simulink model "AC_PCS_mo_2018a"  (R2018b)
settings: Solver=ode4  StartTime=0.0  StopTime=1.2  FixedStep=1e-6  RelTol=1e-3
undefined symbols (not defined in the file): Ion, Lithium
libraries: powerlib x29, powerlib_meascontrol x14, powerlib_extras x6, simulink x4, electricdrivelib x1, re_lib x1
settings Model: Creator=kc  LastModifiedBy=12657

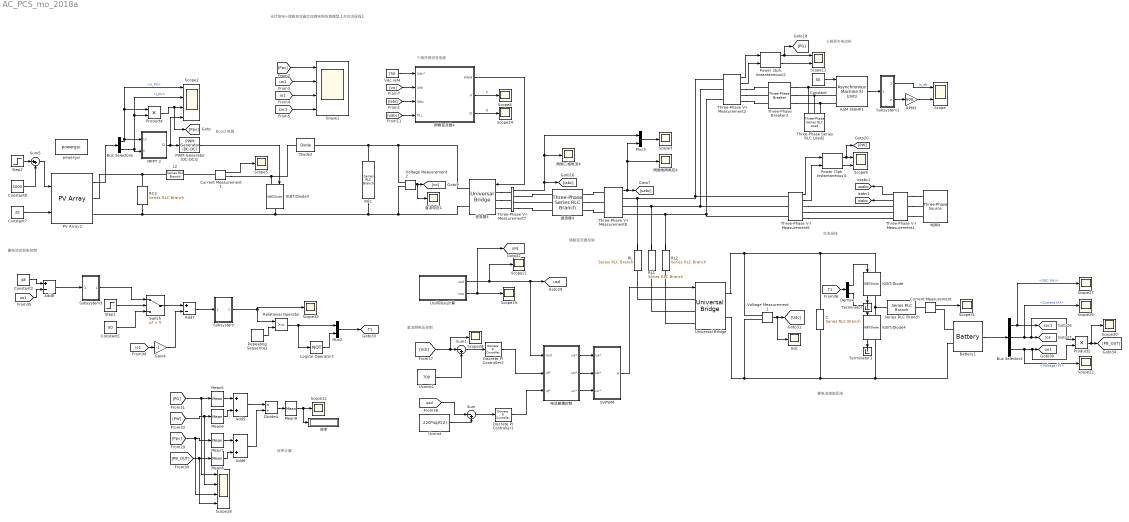
== system AC_PCS_mo_2018a ==
  note: 光伏发电+储能变流器交流微电网仿真模型【共交流母线】
  note: 蓄电池充放电控制
  note: 直流侧电压控制
  note: 三相并网逆变电路
  note: 蓄电池储能系统
  note: 效率计算
  note: 三相异步电动机
  note: 交流母线
  note: 储能变流器控制
  note: Boost 电路
  ASM 350HP1 : powerlib/Machines/Asynchronous Machine SI Units  RotorType=Squirrel-cage  PresetModel=No  MechanicalLoad=Torque Tm  ShowDetailedParameters=on  ReferenceFrame=Rotor  Units=SI  MeasurementBus=off  NominalParameters=[ 2250*746, 400, 50 ]  Stator=[ 0.029 0.226/377]  Rotor=[ 0.022 0.226/377]  Cage1=[ 0.022 0.226/377]  Cage2=[ 0.022 0.226/377]  Lm=13.04/377  Mechanical=[ 63.87 0 2]  PolePairs=2  InitialConditions=[0.00611928 0 556.114 556.114 556.114 -53.9807 -173.981 66.0193]  SimulateSaturation=off  Saturation=[14.03593122, 27.81365428, 53.79336849, 72.68890987, 97.98006896, 148.6815601, 215.7428561, 302.9841135, 428.7778367 ; 230, 322, 414, 460, 506, 552, 598, 644, 690]  LoadFlowParameters=1492000  TsPowergui=0  TsBlock=-1  IterativeModel=Forward Euler  IterativeDiscreteModel=Trapezoidal non iterative  Pmec=1.492e+006
      settings: SourceProductName=Simscape Electrical
  Add5 : Sum
  Add6 : Sum
  Add7 : Sum  Inputs=+-
  Add8 : Sum  Inputs=+-
  Battery1 : electricdrivelib/Extra Sources/Battery  BatType=Lithium-Ion  ShowTempParam=off  ThermalPreset=no  ShowAgeParam=off  NomV=48  NomQ=20  SOC=50  Batt_Tr=0.02  PresetModel=off  MaxQ=20  MinV=36  FullV=52  Dis_rate=8.6957  R=0.024  Normal_OP=18.087  expZone="[51.8585     0.982609]"  current=[6.5 13 32.5]  Units=Time  Tci=20  NomT=20  T2=-30  MaxQ2=4.8  FullV2=7.1  Normal_OP2=5.655  expZone2="[6.58           1]"  Rca=0.6  ti=2000  Dp=0  Neq0=0  Tsim=1e6  Ta1=25  Qeol=5.4*0.9  Reol=0.013333*1.2  Char_age=[2.3478, 3]  Dis_age=[2.3478, 10]  N1=1500  N2=10500  N3=1000  N4=1400  Ta2=45  N5=950
      settings: SourceProductName=Simscape Electrical
  Bus Selector2 : BusSelector  OutputSignals=SOC (%),Current (A),Voltage (V)
  Bus Selector6 : BusSelector  OutputSignals=V_PV,I_PV
  C : powerlib/Elements/Series RLC Branch  LConnTagsString=__new0  RConnTagsString=__new0  BranchType=C  Resistance=0.02  Inductance=4e-3  SetiL0=off  InitialCurrent=0  Capacitance=4e-3  Setx0=on  InitialVoltage=650  Measurements=None
      settings: SourceProductName=Simscape Electrical
  Constant : Constant  Value=50
  Constant1 : Constant  Value=50
  Constant2 : Constant  Value=48
  Constant7 : Constant  Value=25
  Constant8 : Constant  Value=1000
  Current Measurement : powerlib/Measurements/Current Measurement  PhasorSimulation=off  OutputType=Complex  PSBequivalent=0
      settings: SourceProductName=Simscape Electrical
  Current Measurement1 : powerlib/Measurements/Current Measurement  PhasorSimulation=off  OutputType=Complex  PSBequivalent=0
      settings: SourceProductName=Simscape Electrical
  Demux : Demux  Outputs=2
  Diode2 : powerlib/Power Electronics/Diode  Ron=0.001  Lon=0  Vf=0.8  IC=0  UseSnubber=off  Rs=500  Cs=250e-9  Measurements=off
      settings: SourceProductName=Simscape Electrical
  Discrete PI Controller1 : powerlib_extras/Discrete  Control Blocks/Discrete PI Controller  Kp=1.2  Ki=30  Par_Limits=[50000 -50000]  Init=0  Ts=1e-6
  Discrete PI Controller2 : powerlib_extras/Discrete  Control Blocks/Discrete PI Controller  Kp=1.2  Ki=90  Par_Limits=[50000 -50000]  Init=0  Ts=1e-6
  Divide4 : Product  Inputs=*/
  Gain4 : Gain  Gain=-1
  IGBT/Diode : powerlib/Power Electronics/IGBT//Diode  Ron=1e-3  Rs=1e5  Cs=inf  Measurements=on
      settings: SourceProductName=Simscape Electrical
  IGBT/Diode3 : powerlib/Power Electronics/IGBT//Diode  Ron=1e-3  Rs=1e5  Cs=inf  Measurements=off
      settings: SourceProductName=Simscape Electrical
  IGBT/Diode4 : powerlib/Power Electronics/IGBT//Diode  Ron=1e-3  Rs=1e5  Cs=inf  Measurements=on
      settings: SourceProductName=Simscape Electrical
  L2 : powerlib/Elements/Series RLC Branch  LConnTagsString=__new0  RConnTagsString=__new0  BranchType=L  Resistance=1  Inductance=6e-3  SetiL0=off  InitialCurrent=0  Capacitance=2e-4  Setx0=off  InitialVoltage=0  Measurements=None
      settings: SourceProductName=Simscape Electrical
  Logical Operator1 : Logic  Operator=NOT  AllPortsSameDT=off  OutDataTypeStr=boolean
  MPPT 2 : Subsystem  TreatAsAtomicUnit=on
  Mean5 : powerlib_meascontrol/Measurements/Mean  Freq=50  Vinit=0  Ts=1e-6
      settings: SourceProductName=Simscape Electrical
  Mean6 : powerlib_meascontrol/Measurements/Mean  Freq=50  Vinit=0  Ts=1e-6
      settings: SourceProductName=Simscape Electrical
  Mean7 : powerlib_meascontrol/Measurements/Mean  Freq=50  Vinit=10  Ts=1e-6
      settings: SourceProductName=Simscape Electrical
  Mean8 : powerlib_meascontrol/Measurements/Mean  Freq=50  Vinit=10  Ts=1e-6
      settings: SourceProductName=Simscape Electrical
  Mean9 : powerlib_meascontrol/Measurements/Mean  Freq=50  Vinit=10  Ts=1e-6
      settings: SourceProductName=Simscape Electrical
  Mux2 : Mux  Inputs=2
  Mux3 : Mux  Inputs=2
  PV Array2 : re_lib/Solar/PV Array  Npar=5  Nser=10  PlotType=array @ 25 deg.C & specified irradiances  S_vec="[ 1000  500  100 ]"  Temp_C_vec="[ 45 25  ]"  ModuleName=A10Green Technology A10J-M60-230  PlotWhenSelected=off  Pm=230.1288  Ncell=60  Voc=36.42  Isc=8.1  Vm=30.36  Im=7.58  beta_Voc_pc=-0.35901  alpha_Isc_pc=0.097  beta_Voc=-0.13075  alpha_Isc=0.007857  IL=8.1068  I0=2.792e-10  nI=0.98145  Rsh=234.4496  Rs=0.19818  BAL=off  Tc=1e-6  Tfilter=5e-5
      settings: SourceProductName=Simscape Electrical
  PWM Generator (DC-DC)2 : powerlib_meascontrol/Pulse & Signal Generators/PWM Generator (DC-DC)  Fsw=20000  Ts=0
      settings: SourceProductName=Simscape Electrical
  "Power (3ph, Instantaneous)1" : powerlib_meascontrol/Measurements/Power (3ph, Instantaneous)
      settings: SourceProductName=Simscape Electrical
  "Power (3ph, Instantaneous)2" : powerlib_meascontrol/Measurements/Power (3ph, Instantaneous)
      settings: SourceProductName=Simscape Electrical
  Product2 : Product
  Product4 : Product
  RC1 : powerlib/Elements/Series RLC Branch  LConnTagsString=__new0  RConnTagsString=__new0  BranchType=C  Resistance=0.001  Inductance=1e-3  SetiL0=off  InitialCurrent=0  Capacitance=3e-2  Setx0=on  InitialVoltage=750  Measurements=None
      settings: SourceProductName=Simscape Electrical
  RC3 : powerlib/Elements/Series RLC Branch  LConnTagsString=__new0  RConnTagsString=__new0  BranchType=C  Resistance=0.1  Inductance=1e-3  SetiL0=off  InitialCurrent=0  Capacitance=1e-3  Setx0=on  InitialVoltage=300  Measurements=None
      settings: SourceProductName=Simscape Electrical
  RL : powerlib/Elements/Series RLC Branch  LConnTagsString=__new0  RConnTagsString=__new0  BranchType=RL  Resistance=0.02  Inductance=2e-3  SetiL0=off  InitialCurrent=0  Capacitance=1e-6  Setx0=off  InitialVoltage=0  Measurements=None
      settings: SourceProductName=Simscape Electrical
  RL1 : powerlib/Elements/Series RLC Branch  LConnTagsString=__new0  RConnTagsString=__new0  BranchType=RL  Resistance=0.02  Inductance=2e-3  SetiL0=off  InitialCurrent=0  Capacitance=1e-6  Setx0=off  InitialVoltage=0  Measurements=None
      settings: SourceProductName=Simscape Electrical
  RL2 : powerlib/Elements/Series RLC Branch  LConnTagsString=__new0  RConnTagsString=__new0  BranchType=RL  Resistance=0.02  Inductance=2e-3  SetiL0=off  InitialCurrent=0  Capacitance=1e-6  Setx0=off  InitialVoltage=0  Measurements=None
      settings: SourceProductName=Simscape Electrical
  RPM3 : Gain  Gain=500  SaturateOnIntegerOverflow=on  OutDataTypeStr=Inherit: Same as input  ParamDataTypeStr=Inherit: Same as input
  Relational Operator : RelationalOperator  OutDataTypeStr=boolean  RndMeth=Simplest
  Repeating Sequence1 : simulink/Sources/Repeating Sequence  rep_seq_t=[0 0.025e-3 0.05e-3]  rep_seq_y=[0 1 0]
  SVPWM : Subsystem
  Scope : Scope  NumInputPorts=2
  Scope1 : Scope  NumInputPorts=4
  Scope11 : Scope  NumInputPorts=2
  Scope{3,5,8,12,19,21..22,24,27..32} (14 alike) : Scope
  Scope18 : Scope  NumInputPorts=4
  Scope2 : Scope  NumInputPorts=4
  Scope9 : Scope  NumInputPorts=2
  Series RLC Branch : powerlib/Elements/Series RLC Branch  LConnTagsString=__new0  RConnTagsString=__new0  BranchType=L  Resistance=1  Inductance=1e-3  SetiL0=off  InitialCurrent=0  Capacitance=1e-6  Setx0=off  InitialVoltage=0  Measurements=None
      settings: SourceProductName=Simscape Electrical
  Step1 : Step  Time=0  SampleTime=0
  Step2 : Step  Time=2  After=200  SampleTime=0
  Subsystem : Subsystem
      mask Display: disp('PI')
  Subsystem1 : Subsystem
  Subsystem3 : Subsystem
      mask Display: disp('PI')
  Sum : Sum  Inputs=|-+
  Sum1 : Sum  Inputs=|-+
  Sum5 : Sum  Inputs=|++
  Switch : Switch  Criteria=u2 > Threshold
  Terminator : Terminator
  Terminator1 : Terminator
  Three-Phase Series RLC Load2 : powerlib/Elements/Three-Phase Series RLC Load  LConnTagsString=A|B|C  Configuration=Y (grounded)  NominalVoltage=380  Vabc=[1e3 1e3 1e3]  Vabcp=[1e3 1e3 1e3]  NominalFrequency=50  UnbalancedPower=off  ActivePower=5e2  InductivePower=0  CapacitivePower=0  Pabc=[10e3 9e3 11e3]  QLabc=[100 90 110]  QCabc=[100 90 110]  Pabcp=[10e3 9e3 11e3]  QLabcp=[100 90 110]  QCabcp=[100 90 110]  Measurements=None  LoadType=constant Z
      settings: SourceProductName=Simscape Electrical
  Three-Phase V-I Measurement1 : powerlib/Measurements/Three-Phase V-I Measurement  VoltageMeasurement=phase-to-ground  SetLabelV=off  LabelV=Vabc  Vpu=off  VpuLL=off  CurrentMeasurement=yes  SetLabelI=off  LabelI=Iabc  Ipu=off  Pbase=100e6  Vbase=500e3  OutputType=Complex  PhasorSimulation=off  PSBequivalent=0
      settings: SourceProductName=Simscape Electrical
  Three-Phase V-I Measurement2 : powerlib/Measurements/Three-Phase V-I Measurement  VoltageMeasurement=phase-to-ground  SetLabelV=off  LabelV=uabc  Vpu=off  VpuLL=off  CurrentMeasurement=yes  SetLabelI=off  LabelI=iabc1  Ipu=off  Pbase=100e6  Vbase=500e3  OutputType=Complex  PhasorSimulation=off  PSBequivalent=0
      settings: SourceProductName=Simscape Electrical
  Three-Phase V-I Measurement5 : powerlib/Measurements/Three-Phase V-I Measurement  VoltageMeasurement=phase-to-ground  SetLabelV=off  LabelV=Vabc  Vpu=off  VpuLL=off  CurrentMeasurement=yes  SetLabelI=off  LabelI=Iabc  Ipu=off  Pbase=100e6  Vbase=500e3  OutputType=Complex  PhasorSimulation=off  PSBequivalent=0
      settings: SourceProductName=Simscape Electrical
  Three-Phase V-I Measurement7 : powerlib/Measurements/Three-Phase V-I Measurement  VoltageMeasurement=no  SetLabelV=off  LabelV=Vabc  Vpu=off  VpuLL=off  CurrentMeasurement=yes  SetLabelI=off  LabelI=iabc  Ipu=off  Pbase=100e6  Vbase=500e3  OutputType=Complex  PhasorSimulation=off  PSBequivalent=0
      settings: SourceProductName=Simscape Electrical
  Three-Phase V-I Measurement8 : powerlib/Measurements/Three-Phase V-I Measurement  VoltageMeasurement=phase-to-ground  SetLabelV=off  LabelV=uabc  Vpu=off  VpuLL=off  CurrentMeasurement=no  SetLabelI=on  LabelI=iabc1  Ipu=off  Pbase=100e6  Vbase=500e3  OutputType=Complex  PhasorSimulation=off  PSBequivalent=0
      settings: SourceProductName=Simscape Electrical
  Three-Phase Breaker2 : powerlib/Elements/Three-Phase Breaker  InitialState=open  SwitchA=on  SwitchB=on  SwitchC=on  SwitchTimes=[0]  External=off  BreakerResistance=0.01  SnubberResistance=1e6  SnubberCapacitance=inf  Measurements=None
      settings: SourceProductName=Simscape Electrical
  Uconst : Constant  Value=220*sqrt(2)
  Uconst1 : Constant  Value=700
  Udc : Scope
  Universal Bridge : powerlib/Power Electronics/Universal Bridge  Arms=3  SnubberResistance=1e5  SnubberCapacitance=inf  Device=IGBT / Diodes  Ron=1e-3  Lon=0  ForwardVoltages="[  0  0  ]"  ForwardVoltage=0  GTOparameters=[ 10e-6 , 20e-6 ]  IGBTparameters=[ 1e-6 , 2e-6 ]  Measurements=None  Measurements_2=None  converterType=Rectifier
      settings: SourceProductName=Simscape Electrical
  Usd和Usq计算 : Subsystem
  Vdc,ref4 : Constant  Value=750
  Voltage Measurement1 : powerlib/Measurements/Voltage Measurement  PhasorSimulation=off  OutputType=Complex  PSBequivalent=0
      settings: SourceProductName=Simscape Electrical
  Voltage Measurement2 : powerlib/Measurements/Voltage Measurement  PhasorSimulation=off  OutputType=Complex  PSBequivalent=0
      settings: SourceProductName=Simscape Electrical
  powergui : powerlib/powergui  Priority=1  SimulationMode=Discrete  SampleTime=1e-6  frequency=60  Iterations=50  frequencyindice=0  Pbase=100e6  ErrMax=1e-4  UnitsV=kV  UnitsW=MW  buscounter=0  FunctionMessages=off  echomessages=off  EnableUseOfTLC=off  CurrentSourceSwitches=off  DisableSnubberDevices=off  DisableRonSwitches=off  DisableVfSwitches=off  DisplayEquations=off  SolverType=Tustin/Backward Euler (TBE)  Interpol=off  ExternalGateDelay=off  methode=off  Ts=100  x0status=blocks  SPID=on  SwTol=0  HookPort=off  RestoreLinks=warning  ResistiveCurrentMeasurement=off  Frange=[0:2:500]  Ylog=off  Xlog=on  ShowGrid=off  save=off  variable=ZData  structure=0  ZoomFFT=off  StartTime=0.0  cycles=1  DisplayStyle=1  fundamental=60  FreqAxis=off  MaxFrequency=1000  frequencyindicesteady=1  RmsSteady=1  display=off
  效率 : Display
  滤波器4 : powerlib/Elements/Three-Phase Series RLC Branch  LConnTagsString=A|B|C  RConnTagsString=A|B|C  BranchType=RL  Resistance=3/8  Inductance=8e-3  Capacitance=1e-6  Measurements=None
      settings: SourceProductName=Simscape Electrical
  电流解耦控制 : Subsystem
  电网4 : powerlib/Electrical Sources/Three-Phase Source  InternalConnection=Yg  VoltagePhases=off  Voltage=380  PhaseAngle=0  Voltage_phases=[25e3 25e3 25e3]/sqrt(3)  PhaseAngles_phases=[0 -120 +120]  Frequency=50  NonIdealSource=off  SpecifyImpedance=off  Resistance=0.01  Inductance=0  ShortCircuitLevel=100e6  BaseVoltage=25e3  XRratio=7  BusType=swing  Pref=0  Qref=0  Prefabc=[10e3, 10e3, 10e3]  Qrefabc=[0, 0, 0]  Qmin=-inf  Qmax=inf
      settings: SourceProductName=Simscape Electrical
  直流电压1 : Scope
  网侧三相电流4 : Scope
  网侧变流器4 : Subsystem
  网侧电网电压4 : Scope
  逆变器4 : powerlib/Power Electronics/Universal Bridge  Arms=3  SnubberResistance=1e5  SnubberCapacitance=inf  Device=IGBT / Diodes  Ron=1e-3  Lon=0  ForwardVoltages="[  0  0  ]"  ForwardVoltage=0  GTOparameters=[ 10e-6 , 20e-6 ]  IGBTparameters=[ 5e-6 , 5e-6 ]  Measurements=None  Measurements_2=None  converterType=Rectifier
      settings: SourceProductName=Simscape Electrical
  tag scope: T1=global, io1=global, isabc=global, soc1=global, uo1=global, usabc=global, usd=global, usq=global
  wires:
  Three-Phase V-I Measurement8/1 -> Mux3/2, 网侧电网电压4/1, [uabc]
  Mux3/1 -> Scope3/1
  [uabc] -> 网侧变流器4/4(PLL)
  网侧变流器4/2(P) -> Scope8/1  "P"
  网侧变流器4/3(Q) -> Scope24/1  "Q"
  [iabc] -> 网侧变流器4/3(Iabc)
  网侧变流器4/1(PWM) -> 逆变器4/1
  [vo] -> 网侧变流器4/2(Udc)
  Vdc,ref4/1 -> 网侧变流器4/1(Udc*)
  Three-Phase V-I Measurement7/1 -> Mux3/1, 网侧三相电流4/1, [iabc]
  Constant/1 -> ASM 350HP1/1
  Three-Phase V-I Measurement1/1 -> [usabc]
  Three-Phase V-I Measurement1/2 -> [isabc]
  ASM 350HP1/1 -> Subsystem1/1(In1)
  Subsystem1/1(is_ab) -> Scope/1  "is_ab"
  RPM3/1 -> Scope/2
  Subsystem1/2(w) -> RPM3/1
  "Power (3ph, Instantaneous)1"/1 -> [PW], Scope9/1
  "Power (3ph, Instantaneous)1"/2 -> Scope9/2
  Three-Phase V-I Measurement2/1 -> "Power (3ph, Instantaneous)2"/1
  Three-Phase V-I Measurement2/2 -> "Power (3ph, Instantaneous)2"/2
  "Power (3ph, Instantaneous)2"/1 -> [PG], Scope11/1
  "Power (3ph, Instantaneous)2"/2 -> Scope11/2
  Three-Phase V-I Measurement5/1 -> "Power (3ph, Instantaneous)1"/1
  Three-Phase V-I Measurement5/2 -> "Power (3ph, Instantaneous)1"/2
  Add5/1 -> Divide4/1
  Divide4/1 -> Mean9/1
  Add6/1 -> Divide4/2
  Mean5/1 -> Add5/1
  [PG] -> Scope18/1, Mean5/1
  [PW] -> Scope18/2, Mean6/1
  Mean6/1 -> Add5/2
  Mean7/1 -> Add6/1
  [Ppv] -> Scope18/3, Mean7/1
  [PB_OUT] -> Scope18/4, Mean8/1
  Mean8/1 -> Add6/2
  Mean9/1 -> 效率/1, Scope12/1
  [Udc] -> Scope28/1, Sum1/1
  Sum1/1 -> Discrete PI Controller2/1
  Uconst1/1 -> Sum1/2
  Discrete PI Controller2/1 -> 电流解耦控制/2(id*)
  Constant2/1 -> Add8/1
  [io1] -> Gain4/1
  Constant1/1 -> Switch/3
  Gain4/1 -> Add7/2
  Logical Operator1/1 -> Mux2/2
  Switch/1 -> Add7/1
  Mux2/1 -> [T1]
  Subsystem/1(Out1) -> Scope32/1, Relational Operator/1
  Add8/1 -> Subsystem3/1(In1)
  Add7/1 -> Subsystem/1(In1)
  Subsystem3/1(Out1) -> Switch/1
  Repeating Sequence1/1 -> Relational Operator/2
  [uo1] -> Add8/2
  Step1/1 -> Switch/2
  Relational Operator/1 -> Mux2/1, Logical Operator1/1
  Product2/1 -> Scope30/1, [PB_OUT]
  电流解耦控制/2(ub*) -> SVPWM/2(ub*)
  [usd] -> Sum/1
  [T1] -> Demux/1
  Voltage Measurement1/1 -> [Udc], Udc/1
  Demux/2 -> IGBT/Diode4/1
  Demux/1 -> IGBT/Diode/1
  IGBT/Diode4/1 -> Terminator1/1
  Battery1/1 -> Bus Selector2/1
  Bus Selector2/1 -> Scope27/1, [soc1]  "<SOC (%)>"
  Bus Selector2/3 -> Scope22/1, Product2/2, [uo1]  "<Voltage (V)>"
  IGBT/Diode/1 -> Terminator/1
  Discrete PI Controller1/1 -> 电流解耦控制/3(iq*)
  Usd和Usq计算/2(usq) -> [usq], Scope19/1
  Bus Selector2/2 -> Scope29/1, Product2/1, [io1]  "<Current (A)>"
  Uconst/1 -> Sum/2
  电流解耦控制/1(ua*) -> SVPWM/1(ua*)
  Current Measurement/1 -> Scope31/1
  Usd和Usq计算/1(usd) -> [usd], 电流解耦控制/1(Usd), Scope21/1
  电流解耦控制/3(uc*) -> SVPWM/3(uc*)
  SVPWM/1(g) -> Universal Bridge/1
  Sum/1 -> Discrete PI Controller1/1
  [Ppv] -> Scope1/1
  [uo1] -> Scope1/2
  [io1] -> Scope1/3
  [soc1] -> Scope1/4
  Bus Selector6/1 -> Product4/1, Scope2/1, MPPT 2/1("Ui ")  "<V_PV>"
  PWM Generator (DC-DC)2/1 -> IGBT/Diode3/1
  Constant8/1 -> Sum5/2
  PV Array2/1 -> Bus Selector6/1
  Sum5/1 -> PV Array2/1
  Bus Selector6/2 -> Product4/2, Scope2/2, MPPT 2/2("Ii ")  "<I_PV>"
  Step2/1 -> Sum5/1
  Product4/1 -> [Ppv], Scope2/3
  Constant7/1 -> PV Array2/2
  MPPT 2/1(D) -> Scope2/4, PWM Generator (DC-DC)2/1
  Current Measurement1/1 -> Scope5/1
  Voltage Measurement2/1 -> [vo], 直流电压1/1
  connections:
  逆变器4/LConn2 -- Three-Phase V-I Measurement7/LConn2
  逆变器4/LConn3 -- Three-Phase V-I Measurement7/LConn3
  滤波器4/RConn2 -- Three-Phase V-I Measurement8/LConn2
  滤波器4/RConn1 -- Three-Phase V-I Measurement8/LConn1
  Three-Phase V-I Measurement7/RConn1 -- 滤波器4/LConn1
  滤波器4/RConn3 -- Three-Phase V-I Measurement8/LConn3
  逆变器4/LConn1 -- Three-Phase V-I Measurement7/LConn1
  滤波器4/LConn2 -- Three-Phase V-I Measurement7/RConn2
  Three-Phase V-I Measurement7/RConn3 -- 滤波器4/LConn3
  Three-Phase Series RLC Load2/LConn1 -- Three-Phase Breaker2/RConn1 -- ASM 350HP1/LConn1
  Three-Phase Series RLC Load2/LConn2 -- Three-Phase Breaker2/RConn2 -- ASM 350HP1/LConn2
  Three-Phase Series RLC Load2/LConn3 -- ASM 350HP1/LConn3 -- Three-Phase Breaker2/RConn3
  Three-Phase V-I Measurement1/LConn1 -- 电网4/RConn1
  Three-Phase V-I Measurement1/LConn2 -- 电网4/RConn2
  Three-Phase V-I Measurement1/LConn3 -- 电网4/RConn3
  Three-Phase V-I Measurement2/RConn1 -- Three-Phase Breaker2/LConn1
  Three-Phase V-I Measurement2/RConn2 -- Three-Phase Breaker2/LConn2
  Three-Phase V-I Measurement2/RConn3 -- Three-Phase Breaker2/LConn3
  Three-Phase V-I Measurement5/RConn1 -- Three-Phase V-I Measurement1/RConn1
  Three-Phase V-I Measurement5/RConn2 -- Three-Phase V-I Measurement1/RConn2
  Three-Phase V-I Measurement5/RConn3 -- Three-Phase V-I Measurement1/RConn3
  C/RConn1 -- IGBT/Diode4/RConn1 -- Battery1/LConn2 -- Universal Bridge/RConn2 -- Voltage Measurement1/LConn2
  Universal Bridge/RConn1 -- Voltage Measurement1/LConn1 -- C/LConn1 -- IGBT/Diode/LConn1
  IGBT/Diode/RConn1 -- Series RLC Branch/LConn1 -- IGBT/Diode4/LConn1
  Current Measurement/LConn1 -- Series RLC Branch/RConn1
  Battery1/LConn1 -- Current Measurement/RConn1
  Universal Bridge/LConn3 -- RL2/RConn1
  Universal Bridge/LConn2 -- RL1/RConn1
  Universal Bridge/LConn1 -- RL/RConn1
  Three-Phase V-I Measurement8/RConn1 -- Three-Phase V-I Measurement5/LConn1 -- Three-Phase V-I Measurement2/LConn1 -- RL/LConn1
  Three-Phase V-I Measurement8/RConn2 -- Three-Phase V-I Measurement2/LConn2 -- Three-Phase V-I Measurement5/LConn2 -- RL1/LConn1
  RL2/LConn1 -- Three-Phase V-I Measurement2/LConn3 -- Three-Phase V-I Measurement5/LConn3 -- Three-Phase V-I Measurement8/RConn3
  L2/LConn1 -- PV Array2/RConn1 -- RC3/LConn1
  PV Array2/RConn2 -- RC1/RConn1 -- Voltage Measurement2/LConn2 -- 逆变器4/RConn2 -- IGBT/Diode3/RConn1 -- RC3/RConn1
  Current Measurement1/RConn1 -- IGBT/Diode3/LConn1 -- Diode2/LConn1
  RC1/LConn1 -- Diode2/RConn1 -- 逆变器4/RConn1 -- Voltage Measurement2/LConn1
  Current Measurement1/LConn1 -- L2/RConn1

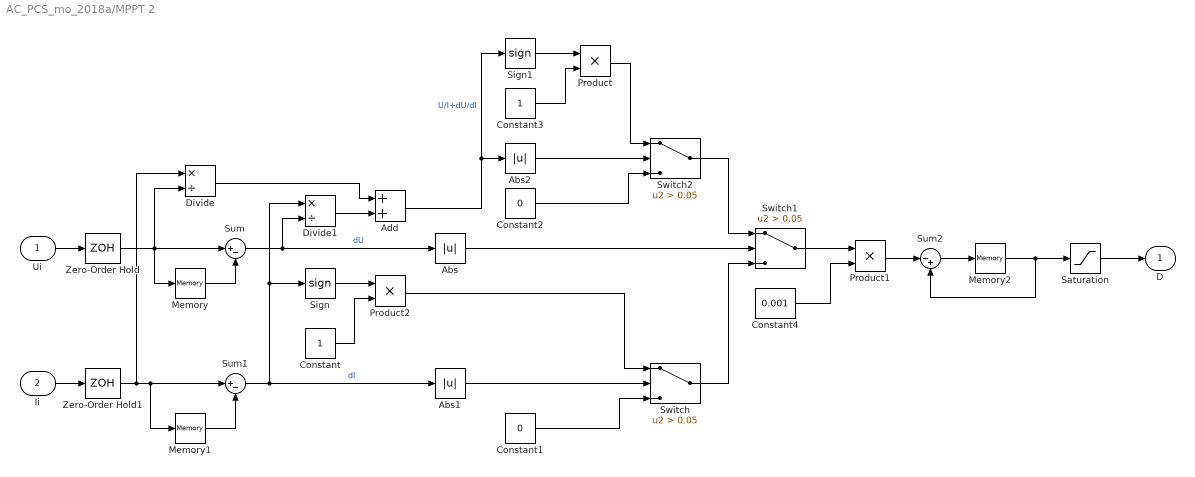
== system AC_PCS_mo_2018a/MPPT 2 ==
  "Ui " : Inport
  "Ii " : Inport  Port=2
  Abs : Abs
  Abs1 : Abs
  Abs2 : Abs
  Add : Sum
  Constant : Constant
  Constant1 : Constant  Value=0
  Constant2 : Constant  Value=0
  Constant3 : Constant
  Constant4 : Constant  Value=0.001
  Divide : Product  Inputs=*/
  Divide1 : Product  Inputs=*/
  Memory : Memory  InheritSampleTime=on
  Memory1 : Memory  InheritSampleTime=on
  Memory2 : Memory  InitialCondition=0.6  InheritSampleTime=on
  Product : Product
  Product1 : Product
  Product2 : Product
  Saturation : Saturate  UpperLimit=1  LowerLimit=0
  Sign : Signum
  Sign1 : Signum
  Sum : Sum  Inputs=|+-
  Sum1 : Sum  Inputs=|+-
  Sum2 : Sum  Inputs=|-+
  Switch : Switch  Criteria=u2 > Threshold  Threshold=0.05
  Switch1 : Switch  Criteria=u2 > Threshold  Threshold=0.05
  Switch2 : Switch  Criteria=u2 > Threshold  Threshold=0.05
  Zero-Order Hold : ZeroOrderHold  SampleTime=0.01
  Zero-Order Hold1 : ZeroOrderHold  SampleTime=0.01
  D : Outport  VectorParamsAs1DForOutWhenUnconnected=on
  wires:
  "Ui "/1 -> Zero-Order Hold/1
  "Ii "/1 -> Zero-Order Hold1/1
  Zero-Order Hold/1 -> Sum/1, Divide/2, Memory/1
  Memory/1 -> Sum/2
  Memory1/1 -> Sum1/2
  Zero-Order Hold1/1 -> Sum1/1, Memory1/1, Divide/1
  Sum/1 -> Divide1/2, Abs/1  "dU"
  Sum1/1 -> Abs1/1, Sign/1, Divide1/1  "dI"
  Divide/1 -> Add/1
  Divide1/1 -> Add/2
  Sign/1 -> Product2/1
  Constant/1 -> Product2/2
  Abs1/1 -> Switch/2
  Constant1/1 -> Switch/3
  Product2/1 -> Switch/1
  Abs/1 -> Switch1/2
  Add/1 -> Abs2/1, Sign1/1  "U/I+dU/dI"
  Abs2/1 -> Switch2/2
  Constant2/1 -> Switch2/3
  Sign1/1 -> Product/1
  Constant3/1 -> Product/2
  Product/1 -> Switch2/1
  Switch2/1 -> Switch1/1
  Switch1/1 -> Product1/1
  Constant4/1 -> Product1/2
  Product1/1 -> Sum2/1
  Sum2/1 -> Memory2/1
  Memory2/1 -> Saturation/1, Sum2/2
  Saturation/1 -> D/1
  Switch/1 -> Switch1/3

== system AC_PCS_mo_2018a/SVPWM ==
  ua* : Inport
  ub* : Inport  Port=2
  uc* : Inport  Port=3
  Demux : Demux  Outputs=3
  Mux2 : Mux  Inputs=3
  Terminator : Terminator
  abc to Alpha-Beta-Zero : powerlib_meascontrol/Transformations/abc to Alpha-Beta-Zero
      settings: SourceProductName=Simscape Electrical
  svpwm1 : Subsystem
  g : Outport
  wires:
  ua*/1 -> Mux2/1
  Mux2/1 -> abc to Alpha-Beta-Zero/1
  ub*/1 -> Mux2/2
  uc*/1 -> Mux2/3
  abc to Alpha-Beta-Zero/1 -> Demux/1
  Demux/1 -> svpwm1/1(Ualfa)
  Demux/2 -> svpwm1/2(Ubeta)
  svpwm1/1(sb) -> g/1
  Demux/3 -> Terminator/1

== system AC_PCS_mo_2018a/Subsystem ==
  In1 : Inport
  Add1 : Sum
  Gain : Gain  Gain=20
  Gain1 : Gain  Gain=8
  Integrator : Integrator
  Out1 : Outport
  wires:
  In1/1 -> Gain1/1, Gain/1
  Gain1/1 -> Integrator/1
  Integrator/1 -> Add1/2
  Add1/1 -> Out1/1
  Gain/1 -> Add1/1

== system AC_PCS_mo_2018a/Subsystem1 ==
  In1 : Inport
  Bus Selector1 : BusSelector  OutputSignals=Stator measurements.Stator current is_a (A),Stator measurements.Stator current is_b (A),Stator measurements.Stator current is_c (A),Mechanical.Rotor speed (wm)
  Mux : Mux  Inputs=3
  rad/s to : Gain  Gain=60/2/pi  SaturateOnIntegerOverflow=on  OutDataTypeStr=Inherit: Same as input  ParamDataTypeStr=Inherit: Same as input
  is_ab : Outport  VectorParamsAs1DForOutWhenUnconnected=on
  w : Outport  Port=2  VectorParamsAs1DForOutWhenUnconnected=on
  wires:
  rad/s to/1 -> w/1  "Speed (rpm)"
  In1/1 -> Bus Selector1/1
  Bus Selector1/4 -> rad/s to/1  "<Rotor speed (wm)>"
  Bus Selector1/1 -> Mux/1  "<Stator current is_a (A)>"
  Bus Selector1/2 -> Mux/2  "<Stator current is_b (A)>"
  Bus Selector1/3 -> Mux/3  "<Stator current is_c (A)>"
  Mux/1 -> is_ab/1

== system AC_PCS_mo_2018a/Subsystem3 ==
  In1 : Inport
  Add5 : Sum
  Gain1 : Gain  Gain=10
  Gain5 : Gain  Gain=200
  Integrator2 : Integrator
  Out1 : Outport
  wires:
  Add5/1 -> Out1/1
  Gain1/1 -> Add5/1
  In1/1 -> Gain1/1, Gain5/1
  Gain5/1 -> Integrator2/1
  Integrator2/1 -> Add5/2

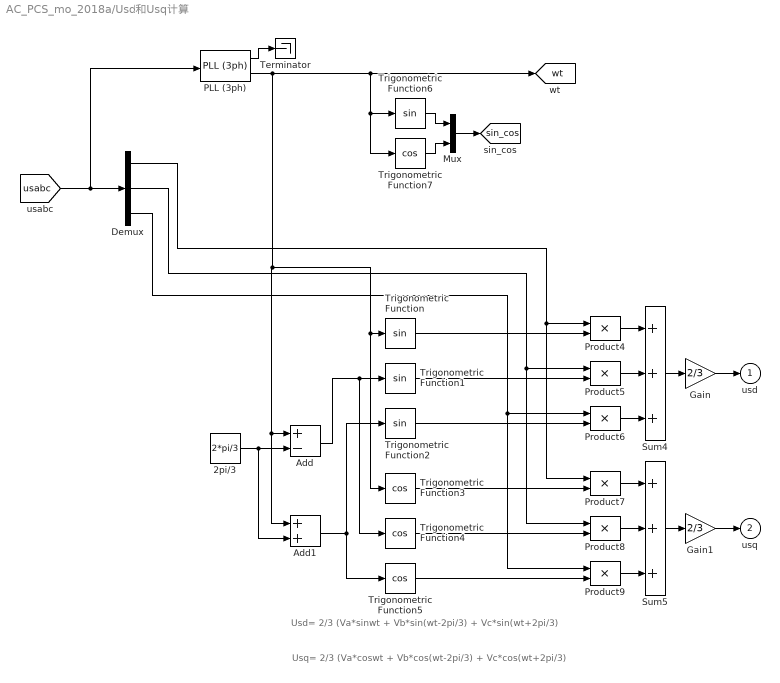
== system AC_PCS_mo_2018a/Usd和Usq计算 ==
  note: Usq= 2/3 (Va*coswt + Vb*cos(wt-2pi/3) + Vc*cos(wt+2pi/3)
  note: Usd= 2/3 (Va*sinwt + Vb*sin(wt-2pi/3) + Vc*sin(wt+2pi/3)
  2pi/3 : Constant  Value=2*pi/3
  Add : Sum  Inputs=+-
  Add1 : Sum
  Demux : Demux  Outputs=3
  Gain : Gain  Gain=2/3
  Gain1 : Gain  Gain=2/3
  Mux : Mux  Inputs=2
  PLL (3ph) : powerlib_meascontrol/PLL/PLL (3ph)  Fmin=45  Par_Init=[0, 50]  ParK=[180, 3200, 1]  TcD=1e-4  MaxRateChangeFreq=12  FilterCutOffFreq=25  Ts=1e-6  AGC=on
      settings: SourceProductName=Simscape Electrical
  Product{4..9} (6 alike) : Product  SaturateOnIntegerOverflow=on  InputSameDT=on  OutDataTypeStr=Inherit: Same as first input
  Sum4 : Sum  Inputs=+++  SaturateOnIntegerOverflow=on  InputSameDT=on  OutDataTypeStr=Inherit: Same as first input
  Sum5 : Sum  Inputs=+++  SaturateOnIntegerOverflow=on  InputSameDT=on  OutDataTypeStr=Inherit: Same as first input
  Terminator : Terminator
  Trigonometric Function{,1..2,6} (4 alike) : Trigonometry
  Trigonometric Function{3..5,7} (4 alike) : Trigonometry  Operator=cos
  usd : Outport  InitialOutput=0
  usq : Outport  Port=2  InitialOutput=0
  tag scope: sin_cos=global, wt=global
  wires:
  Mux/1 -> [sin_cos]
  PLL (3ph)/2 -> Add1/1, Add/1, Trigonometric Function/1, Trigonometric Function3/1, Trigonometric Function7/1, Trigonometric Function6/1, [wt]
  Trigonometric Function5/1 -> Product9/2
  Trigonometric Function4/1 -> Product8/2
  Trigonometric Function3/1 -> Product7/2
  Demux/3 -> Product6/1, Product9/1
  Trigonometric Function2/1 -> Product6/2
  Add1/1 -> Trigonometric Function2/1, Trigonometric Function5/1
  Demux/2 -> Product5/1, Product8/1
  Trigonometric Function1/1 -> Product5/2
  Add/1 -> Trigonometric Function1/1, Trigonometric Function4/1
  Trigonometric Function/1 -> Product4/2
  2pi/3/1 -> Add/2, Add1/2
  Sum5/1 -> Gain1/1
  Product8/1 -> Sum5/2
  Product9/1 -> Sum5/3
  Product7/1 -> Sum5/1
  Sum4/1 -> Gain/1
  Product4/1 -> Sum4/1
  Product6/1 -> Sum4/3
  Product5/1 -> Sum4/2
  Demux/1 -> Product4/1, Product7/1
  [usabc] -> PLL (3ph)/1, Demux/1
  PLL (3ph)/1 -> Terminator/1
  Trigonometric Function6/1 -> Mux/1
  Trigonometric Function7/1 -> Mux/2
  Gain/1 -> usd/1
  Gain1/1 -> usq/1

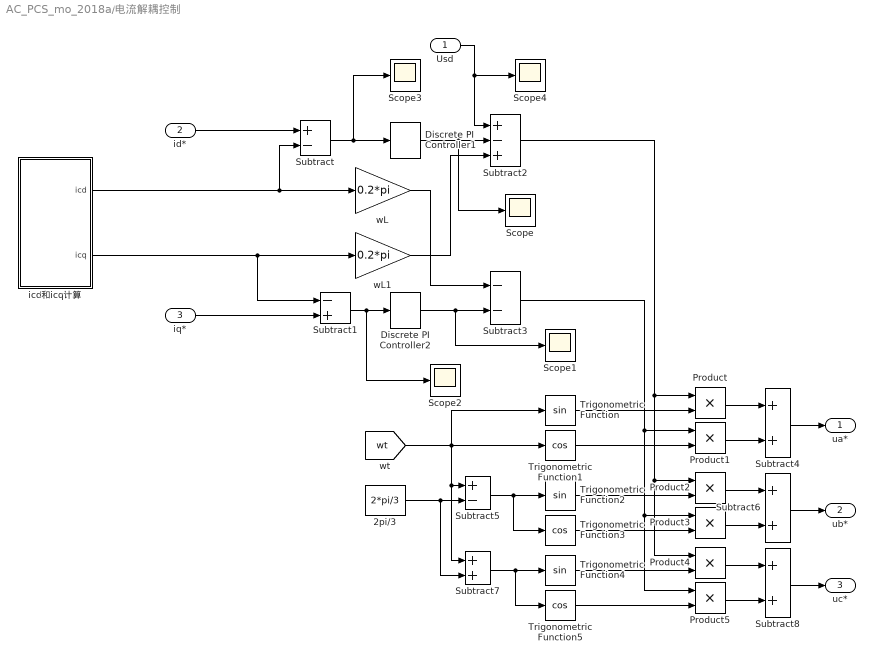
== system AC_PCS_mo_2018a/电流解耦控制 ==
  Usd : Inport
  id* : Inport  Port=2
  iq* : Inport  Port=3
  2pi/3 : Constant  Value=2*pi/3
  Discrete PI Controller1 : powerlib_extras/Discrete  Control Blocks/Discrete PI Controller  Kp=1000  Ki=2000  Par_Limits="[30000  -30000]"  Init=0  Ts=1e-6
  Discrete PI Controller2 : powerlib_extras/Discrete  Control Blocks/Discrete PI Controller  Kp=1000  Ki=2000  Par_Limits="[30000  -30000]"  Init=0  Ts=1e-6
  Product{,1..5} (6 alike) : Product
  Scope{,1..4} (5 alike) : Scope
  Subtract : Sum  Inputs=+-
  Subtract1 : Sum  Inputs=-+
  Subtract2 : Sum  Inputs=+-+
  Subtract3 : Sum  Inputs=--
  Subtract{4,6..8} (4 alike) : Sum
  Subtract5 : Sum  Inputs=+-
  Trigonometric Function : Trigonometry
  Trigonometric Function1 : Trigonometry  Operator=cos
  Trigonometric Function2 : Trigonometry
  Trigonometric Function3 : Trigonometry  Operator=cos
  Trigonometric Function4 : Trigonometry
  Trigonometric Function5 : Trigonometry  Operator=cos
  icd和icq计算 : Subsystem
  wL : Gain  Gain=0.2*pi
  wL1 : Gain  Gain=0.2*pi
  ua* : Outport
  ub* : Outport  Port=2
  uc* : Outport  Port=3
  wires:
  Subtract1/1 -> Discrete PI Controller2/1, Scope2/1
  Usd/1 -> Scope4/1, Subtract2/1
  wL1/1 -> Subtract2/3
  Discrete PI Controller2/1 -> Subtract3/2, Scope1/1
  Product1/1 -> Subtract4/2
  Discrete PI Controller1/1 -> Subtract2/2, Scope/1
  wL/1 -> Subtract3/1
  Subtract6/1 -> ub*/1
  Subtract/1 -> Discrete PI Controller1/1, Scope3/1
  Product5/1 -> Subtract8/2
  Product/1 -> Subtract4/1
  Product3/1 -> Subtract6/2
  Trigonometric Function4/1 -> Product4/2
  icd和icq计算/1(icd) -> Subtract/2, wL/1
  Subtract7/1 -> Trigonometric Function4/1, Trigonometric Function5/1
  Product4/1 -> Subtract8/1
  Subtract2/1 -> Product/1, Product4/1, Product2/1
  Subtract8/1 -> uc*/1
  Product2/1 -> Subtract6/1
  Subtract5/1 -> Trigonometric Function2/1, Trigonometric Function3/1
  2pi/3/1 -> Subtract5/2, Subtract7/2
  Subtract3/1 -> Product5/1, Product3/1, Product1/1
  Trigonometric Function1/1 -> Product1/2
  Subtract4/1 -> ua*/1
  Trigonometric Function2/1 -> Product2/2
  Trigonometric Function5/1 -> Product5/2
  [wt] -> Subtract5/1, Subtract7/1, Trigonometric Function1/1, Trigonometric Function/1
  Trigonometric Function3/1 -> Product3/2
  Trigonometric Function/1 -> Product/2
  icd和icq计算/2(icq) -> Subtract1/1, wL1/1
  id*/1 -> Subtract/1
  iq*/1 -> Subtract1/2

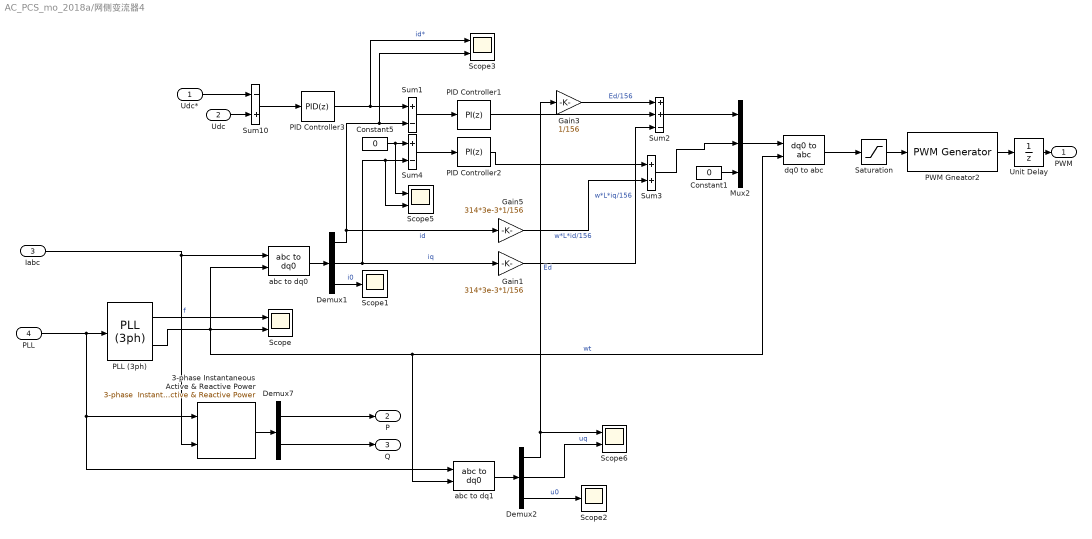
== system AC_PCS_mo_2018a/网侧变流器4 ==
  Udc* : Inport
  Udc : Inport  Port=2
  Iabc : Inport  Port=3
  PLL : Inport  Port=4
  3-phase Instantaneous Active & Reactive Power : powerlib_extras/Measurements/3-phase  Instantaneous  Active & Reactive Power
  Constant1 : Constant  Value=0
  Constant5 : Constant  Value=0
  Demux1 : Demux  Outputs=3
  Demux2 : Demux  Outputs=3
  Demux7 : Demux  Outputs=2
  Gain1 : Gain  Gain=314*3e-3*1/156
  Gain3 : Gain  Gain=1/156
  Gain5 : Gain  Gain=314*3e-3*1/156
  Mux2 : Mux  Inputs=3
  PID Controller1 : simulink/Continuous/PID Controller  Controller=PI  Form=Parallel  TimeDomain=Discrete-time  SampleTime=1e-6  IntegratorMethod=Trapezoidal  FilterMethod=Forward Euler  ControllerParametersSource=internal  P=0.16  I=20  D=0  UseFilter=on  N=100  TunerSelectOption=Transfer Function Based (PID Tuner App)  InitialConditionSource=internal  InitialConditionForIntegrator=0  InitialConditionForFilter=0  DifferentiatorICPrevScaledInput=0  ExternalReset=none  TrackingMode=off  Kt=1  LimitOutput=on  UpperSaturationLimit=6  LowerSaturationLimit=-6  LinearizeAsGain=on  AntiWindupMode=none  Kb=1  POutMin=[]  POutMax=[]  IOutMin=[]  IOutMax=[]  DOutMin=[]  DOutMax=[]  NOutMin=[]  NOutMax=[]  SumOutMin=[]  SumOutMax=[]  SaturationOutMin=[]  SaturationOutMax=[]  PParamMin=[]  PParamMax=[]  IParamMin=[]  IParamMax=[]  DParamMin=[]  DParamMax=[]  NParamMin=[]  NParamMax=[]  KbParamMin=[]  KbParamMax=[]  KtParamMin=[]  KtParamMax=[]  KbOutMin=[]  KbOutMax=[]  KtOutMin=[]  KtOutMax=[]  IntegratorOutMin=[]  IntegratorOutMax=[]  FilterOutMin=[]  FilterOutMax=[]  SumI1OutMin=[]  SumI1OutMax=[]  SumI2OutMin=[]  SumI2OutMax=[]  SumI3OutMin=[]  SumI3OutMax=[]  SumI4OutMin=[]  SumI4OutMax=[]  SumDOutMin=[]  SumDOutMax=[]  DifferentiatorOutMin=[]  DifferentiatorOutMax=[]  FilterDiffOutCoefMin=[]  FilterDiffOutCoefMax=[]  ReciprocalOutMin=[]  ReciprocalOutMax=[]  SumDenOutMin=[]  SumDenOutMax=[]  SumNumOutMin=[]  SumNumOutMax=[]  DivideOutMin=[]  DivideOutMax=[]  IntegratorContinuousStateAttributes=''  IntegratorStateMustResolveToSignalObject=off  IntegratorRTWStateStorageClass=Auto  FilterContinuousStateAttributes=''  FilterStateMustResolveToSignalObject=off  FilterRTWStateStorageClass=Auto  ParallelPVariant=InternalParameters  IdealPVariant=Disabled  IVariant=InternalParameters  DVariant=Disabled  IntegratorVariant=Discrete  SatVariant=Enabled  AWVariant=Passthrough  PCopyVariant=Disabled  TRVariant=Disabled  FdbkBlocksVariant=Forward  IdealPFdbkVariant=Disabled  SatFdbkVariant=Disabled  DerivativeFilterVariant=Disabled  NVariant=Disabled  NCopyVariant=Disabled_SignalSpec  FilterICVariant=Disabled  IntegratorICVariant=InternalICs  ExternalResetVariant=Disabled  TRSumVariant=Passthrough  SumFdbkVariant=Disabled  SumVariant=Sum_PI
  PID Controller2 : simulink/Continuous/PID Controller  Controller=PI  Form=Parallel  TimeDomain=Discrete-time  SampleTime=1e-6  IntegratorMethod=Trapezoidal  FilterMethod=Forward Euler  ControllerParametersSource=internal  P=0.16  I=20  D=0  UseFilter=on  N=100  TunerSelectOption=Transfer Function Based (PID Tuner App)  InitialConditionSource=internal  InitialConditionForIntegrator=0  InitialConditionForFilter=0  DifferentiatorICPrevScaledInput=0  ExternalReset=none  TrackingMode=off  Kt=1  LimitOutput=on  UpperSaturationLimit=6  LowerSaturationLimit=-6  LinearizeAsGain=on  AntiWindupMode=none  Kb=1  POutMin=[]  POutMax=[]  IOutMin=[]  IOutMax=[]  DOutMin=[]  DOutMax=[]  NOutMin=[]  NOutMax=[]  SumOutMin=[]  SumOutMax=[]  SaturationOutMin=[]  SaturationOutMax=[]  PParamMin=[]  PParamMax=[]  IParamMin=[]  IParamMax=[]  DParamMin=[]  DParamMax=[]  NParamMin=[]  NParamMax=[]  KbParamMin=[]  KbParamMax=[]  KtParamMin=[]  KtParamMax=[]  KbOutMin=[]  KbOutMax=[]  KtOutMin=[]  KtOutMax=[]  IntegratorOutMin=[]  IntegratorOutMax=[]  FilterOutMin=[]  FilterOutMax=[]  SumI1OutMin=[]  SumI1OutMax=[]  SumI2OutMin=[]  SumI2OutMax=[]  SumI3OutMin=[]  SumI3OutMax=[]  SumI4OutMin=[]  SumI4OutMax=[]  SumDOutMin=[]  SumDOutMax=[]  DifferentiatorOutMin=[]  DifferentiatorOutMax=[]  FilterDiffOutCoefMin=[]  FilterDiffOutCoefMax=[]  ReciprocalOutMin=[]  ReciprocalOutMax=[]  SumDenOutMin=[]  SumDenOutMax=[]  SumNumOutMin=[]  SumNumOutMax=[]  DivideOutMin=[]  DivideOutMax=[]  IntegratorContinuousStateAttributes=''  IntegratorStateMustResolveToSignalObject=off  IntegratorRTWStateStorageClass=Auto  FilterContinuousStateAttributes=''  FilterStateMustResolveToSignalObject=off  FilterRTWStateStorageClass=Auto  ParallelPVariant=InternalParameters  IdealPVariant=Disabled  IVariant=InternalParameters  DVariant=Disabled  IntegratorVariant=Discrete  SatVariant=Enabled  AWVariant=Passthrough  PCopyVariant=Disabled  TRVariant=Disabled  FdbkBlocksVariant=Forward  IdealPFdbkVariant=Disabled  SatFdbkVariant=Disabled  DerivativeFilterVariant=Disabled  NVariant=Disabled  NCopyVariant=Disabled_SignalSpec  FilterICVariant=Disabled  IntegratorICVariant=InternalICs  ExternalResetVariant=Disabled  TRSumVariant=Passthrough  SumFdbkVariant=Disabled  SumVariant=Sum_PI
  PID Controller3 : simulink/Continuous/PID Controller  Controller=PID  Form=Parallel  TimeDomain=Discrete-time  SampleTime=1e-6  IntegratorMethod=Forward Euler  FilterMethod=Trapezoidal  ControllerParametersSource=internal  P=10  I=100  D=0.1  UseFilter=on  N=100  TunerSelectOption=Transfer Function Based (PID Tuner App)  InitialConditionSource=internal  InitialConditionForIntegrator=0  InitialConditionForFilter=0  DifferentiatorICPrevScaledInput=0  ExternalReset=none  TrackingMode=off  Kt=1  LimitOutput=on  UpperSaturationLimit=500  LowerSaturationLimit=-100  LinearizeAsGain=on  AntiWindupMode=none  Kb=1  POutMin=[]  POutMax=[]  IOutMin=[]  IOutMax=[]  DOutMin=[]  DOutMax=[]  NOutMin=[]  NOutMax=[]  SumOutMin=[]  SumOutMax=[]  SaturationOutMin=[]  SaturationOutMax=[]  PParamMin=[]  PParamMax=[]  IParamMin=[]  IParamMax=[]  DParamMin=[]  DParamMax=[]  NParamMin=[]  NParamMax=[]  KbParamMin=[]  KbParamMax=[]  KtParamMin=[]  KtParamMax=[]  KbOutMin=[]  KbOutMax=[]  KtOutMin=[]  KtOutMax=[]  IntegratorOutMin=[]  IntegratorOutMax=[]  FilterOutMin=[]  FilterOutMax=[]  SumI1OutMin=[]  SumI1OutMax=[]  SumI2OutMin=[]  SumI2OutMax=[]  SumI3OutMin=[]  SumI3OutMax=[]  SumI4OutMin=[]  SumI4OutMax=[]  SumDOutMin=[]  SumDOutMax=[]  DifferentiatorOutMin=[]  DifferentiatorOutMax=[]  FilterDiffOutCoefMin=[]  FilterDiffOutCoefMax=[]  ReciprocalOutMin=[]  ReciprocalOutMax=[]  SumDenOutMin=[]  SumDenOutMax=[]  SumNumOutMin=[]  SumNumOutMax=[]  DivideOutMin=[]  DivideOutMax=[]  IntegratorContinuousStateAttributes=''  IntegratorStateMustResolveToSignalObject=off  IntegratorRTWStateStorageClass=Auto  FilterContinuousStateAttributes=''  FilterStateMustResolveToSignalObject=off  FilterRTWStateStorageClass=Auto  ParallelPVariant=InternalParameters  IdealPVariant=Disabled  IVariant=InternalParameters  DVariant=InternalParameters  IntegratorVariant=Discrete  SatVariant=Enabled  AWVariant=Passthrough  PCopyVariant=Disabled  TRVariant=Disabled  FdbkBlocksVariant=Forward  IdealPFdbkVariant=Disabled  SatFdbkVariant=Disabled  DerivativeFilterVariant=TrapezoidalFilter  NVariant=InternalParameters  NCopyVariant=InternalParameters  FilterICVariant=InternalICsFilter  IntegratorICVariant=InternalICs  ExternalResetVariant=Disabled  TRSumVariant=Passthrough  SumFdbkVariant=Disabled  SumVariant=Sum_PID
  PLL (3ph) : powerlib_meascontrol/PLL/PLL (3ph)  Fmin=45  Par_Init=[0,50]  ParK=[0.2,8]  TcD=1e-4  MaxRateChangeFreq=12  FilterCutOffFreq=25  Ts=5e-5  AGC=on
      settings: SourceProductName=Simscape Electrical
  PWM Gneator2 : powerlib_extras/Control  Blocks/PWM Generator  GeneratorMode="3-arm  bridge (6 pulses)"  Fc=10000  Internal=off  mIndex=0.8  Freq=50  Phase=0
  Saturation : Saturate  UpperLimit=156  LowerLimit=-156
  Scope{,3,5..6} (4 alike) : Scope  NumInputPorts=2
  Scope1 : Scope
  Scope2 : Scope
  Sum1 : Sum  Inputs=+-
  Sum10 : Sum  Inputs=-+
  Sum2 : Sum  Inputs=++-
  Sum3 : Sum
  Sum4 : Sum  Inputs=+-
  Unit Delay : UnitDelay  SampleTime=-1
  abc to dq0 : powerlib_meascontrol/Transformations/abc to dq0  Alignment=90 degrees behind phase A axis
      settings: SourceProductName=Simscape Electrical
  abc to dq1 : powerlib_meascontrol/Transformations/abc to dq0  Alignment=90 degrees behind phase A axis
      settings: SourceProductName=Simscape Electrical
  dq0 to abc : powerlib_meascontrol/Transformations/dq0 to abc  Alignment=90 degrees behind phase A axis
      settings: SourceProductName=Simscape Electrical
  PWM : Outport
  P : Outport  Port=2
  Q : Outport  Port=3
  wires:
  Unit Delay/1 -> PWM/1
  PWM Gneator2/1 -> Unit Delay/1
  Udc/1 -> Sum10/2
  Udc*/1 -> Sum10/1
  PID Controller3/1 -> Scope3/1, Sum1/1  "id*"
  Sum10/1 -> PID Controller3/1
  Iabc/1 -> abc to dq0/1, 3-phase Instantaneous Active & Reactive Power/2
  Sum4/1 -> PID Controller2/1
  Sum1/1 -> PID Controller1/1
  PLL/1 -> PLL (3ph)/1, abc to dq1/1, 3-phase Instantaneous Active & Reactive Power/1
  abc to dq0/1 -> Demux1/1
  Constant5/1 -> Scope5/1, Sum4/1
  Demux1/2 -> Gain1/1, Scope5/2, Sum4/2  "iq"
  Constant1/1 -> Mux2/3
  PLL (3ph)/2 -> dq0 to abc/2, abc to dq1/2, Scope/2, abc to dq0/2  "wt"
  3-phase Instantaneous Active & Reactive Power/1 -> Demux7/1
  Demux7/1 -> P/1
  Demux7/2 -> Q/1
  Saturation/1 -> PWM Gneator2/1
  PID Controller1/1 -> Sum2/2
  PID Controller2/1 -> Sum3/1
  Demux1/1 -> Gain5/1, Scope3/2, Sum1/2  "id"
  Gain1/1 -> Sum2/3  "w*L*iq/156"
  abc to dq1/1 -> Demux2/1
  Demux2/1 -> Scope6/1, Gain3/1  "Ed"
  Demux2/2 -> Scope6/2  "uq"
  Sum3/1 -> Mux2/2
  Sum2/1 -> Mux2/1
  Gain3/1 -> Sum2/1  "Ed/156"
  PLL (3ph)/1 -> Scope/1  "f"
  Demux1/3 -> Scope1/1  "i0"
  Demux2/3 -> Scope2/1  "u0"
  Mux2/1 -> dq0 to abc/1
  dq0 to abc/1 -> Saturation/1
  Gain5/1 -> Sum3/2  "w*L*id/156"

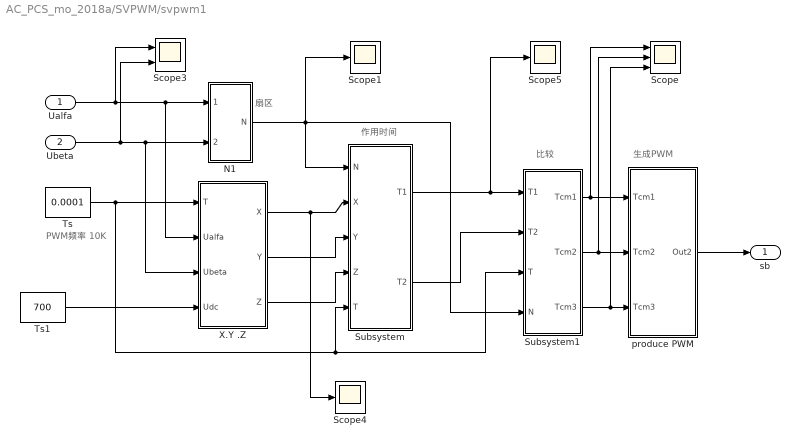
== system AC_PCS_mo_2018a/SVPWM/svpwm1 ==
  note: PWM频率
      | 10K
  note: 生成PWM
  note: 比较
  note: 作用时间
  note: 扇区
  Ualfa : Inport
  Ubeta : Inport  Port=2
  N1 : Subsystem
  Scope : Scope  NumInputPorts=3
  Scope1 : Scope
  Scope3 : Scope  NumInputPorts=2
  Scope4 : Scope
  Scope5 : Scope
  Subsystem : Subsystem
  Subsystem1 : Subsystem
  Ts : Constant  Value=0.0001
  Ts1 : Constant  Value=700
  X.Y .Z : Subsystem
  produce PWM : Subsystem
  sb : Outport
  wires:
  Ts/1 -> X.Y .Z/1(T), Subsystem1/3(T), Subsystem/5(T)
  Ts1/1 -> X.Y .Z/4(Udc)
  N1/1(N) -> Subsystem/1(N), Subsystem1/4(N), Scope1/1
  X.Y .Z/1(X) -> Subsystem/2(X), Scope4/1
  X.Y .Z/2(Y) -> Subsystem/3(Y)
  X.Y .Z/3(Z) -> Subsystem/4(Z)
  Subsystem1/1(Tcm1) -> produce PWM/1(Tcm1), Scope/1
  Subsystem1/2(Tcm2) -> Scope/2, produce PWM/2(Tcm2)
  Subsystem1/3(Tcm3) -> Scope/3, produce PWM/3(Tcm3)
  Ualfa/1 -> Scope3/1, X.Y .Z/2(Ualfa), N1/1(Ualfa)
  Subsystem/1(T1) -> Scope5/1, Subsystem1/1(T1)
  Subsystem/2(T2) -> Subsystem1/2(T2)
  Ubeta/1 -> N1/2(Ubeta), X.Y .Z/3(Ubeta), Scope3/2
  produce PWM/1(Out2) -> sb/1

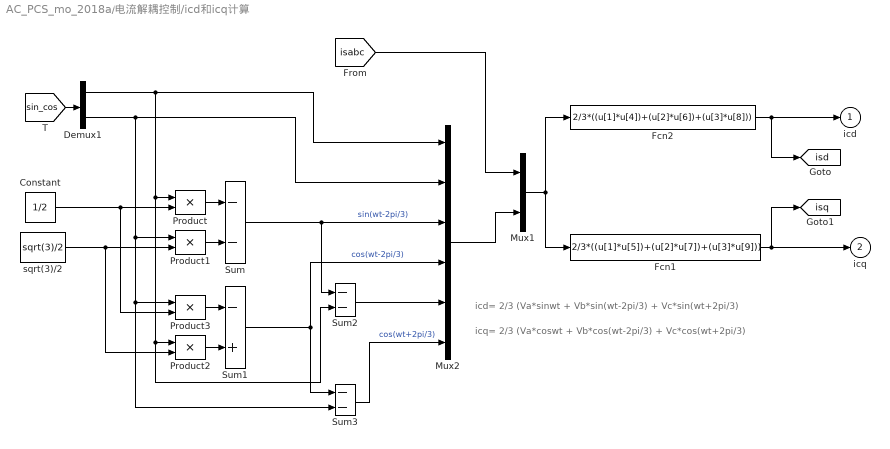
== system AC_PCS_mo_2018a/电流解耦控制/icd和icq计算 ==
  note: icq= 2/3 (Va*coswt + Vb*cos(wt-2pi/3) + Vc*cos(wt+2pi/3)
  note: icd= 2/3 (Va*sinwt + Vb*sin(wt-2pi/3) + Vc*sin(wt+2pi/3)
  Constant : Constant  Value=1/2
  Demux1 : Demux  Outputs=2
  Fcn1 : Fcn  Expr=2/3*((u[1]*u[5])+(u[2]*u[7])+(u[3]*u[9]))
  Fcn2 : Fcn  Expr=2/3*((u[1]*u[4])+(u[2]*u[6])+(u[3]*u[8]))
  Mux1 : Mux  Inputs=2
  Mux2 : Mux  Inputs=6
  Product{,1..3} (4 alike) : Product  SaturateOnIntegerOverflow=on  InputSameDT=on  OutDataTypeStr=Inherit: Same as first input
  Sum : Sum  Inputs=--  SaturateOnIntegerOverflow=on  InputSameDT=on  OutDataTypeStr=Inherit: Same as first input
  Sum1 : Sum  Inputs=-+  SaturateOnIntegerOverflow=on  InputSameDT=on  OutDataTypeStr=Inherit: Same as first input
  Sum2 : Sum  Inputs=--  SaturateOnIntegerOverflow=on  InputSameDT=on  OutDataTypeStr=Inherit: Same as first input
  Sum3 : Sum  Inputs=--  SaturateOnIntegerOverflow=on  InputSameDT=on  OutDataTypeStr=Inherit: Same as first input
  sqrt(3)/2 : Constant  Value=sqrt(3)/2
  icd : Outport  InitialOutput=0
  icq : Outport  Port=2  InitialOutput=0
  tag scope: isd=global, isq=global
  wires:
  Product/1 -> Sum/1
  Sum/1 -> Sum2/1, Mux2/3  "sin(wt-2pi/3)"
  Product1/1 -> Sum/2
  Sum2/1 -> Mux2/5
  Sum3/1 -> Mux2/6  "cos(wt+2pi/3)"
  Mux2/1 -> Mux1/2
  Sum1/1 -> Sum3/1, Mux2/4  "cos(wt-2pi/3)"
  Demux1/1 -> Mux2/1, Sum2/2, Product2/1, Product/1
  Product2/1 -> Sum1/2
  Product3/1 -> Sum1/1
  [sin_cos] -> Demux1/1
  Constant/1 -> Product3/2, Product/2
  sqrt(3)/2/1 -> Product2/2, Product1/2
  Mux1/1 -> Fcn1/1, Fcn2/1
  Demux1/2 -> Product1/1, Product3/1, Sum3/2, Mux2/2
  [isabc] -> Mux1/1
  Fcn2/1 -> [isd], icd/1
  Fcn1/1 -> [isq], icq/1

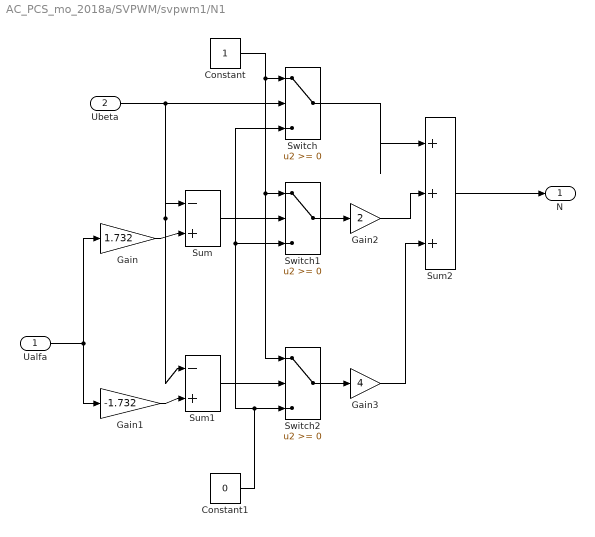
== system AC_PCS_mo_2018a/SVPWM/svpwm1/N1 ==
  Ualfa : Inport
  Ubeta : Inport  Port=2
  Constant : Constant
  Constant1 : Constant  Value=0
  Gain : Gain  Gain=1.732
  Gain1 : Gain  Gain=-1.732
  Gain2 : Gain  Gain=2
  Gain3 : Gain  Gain=4
  Sum : Sum  Inputs=|-+
  Sum1 : Sum  Inputs=|-+
  Sum2 : Sum  Inputs=|+++
  Switch : Switch
  Switch1 : Switch
  Switch2 : Switch
  N : Outport
  wires:
  Ubeta/1 -> Switch/2, Sum/1, Sum1/1
  Constant/1 -> Switch/1, Switch2/1, Switch1/1
  Ualfa/1 -> Gain1/1, Gain/1
  Gain/1 -> Sum/2
  Sum/1 -> Switch1/2
  Sum1/1 -> Switch2/2
  Gain1/1 -> Sum1/2
  Constant1/1 -> Switch/3, Switch1/3, Switch2/3
  Switch1/1 -> Gain2/1
  Switch2/1 -> Gain3/1
  Gain2/1 -> Sum2/2
  Switch/1 -> Sum2/1
  Gain3/1 -> Sum2/3
  Sum2/1 -> N/1

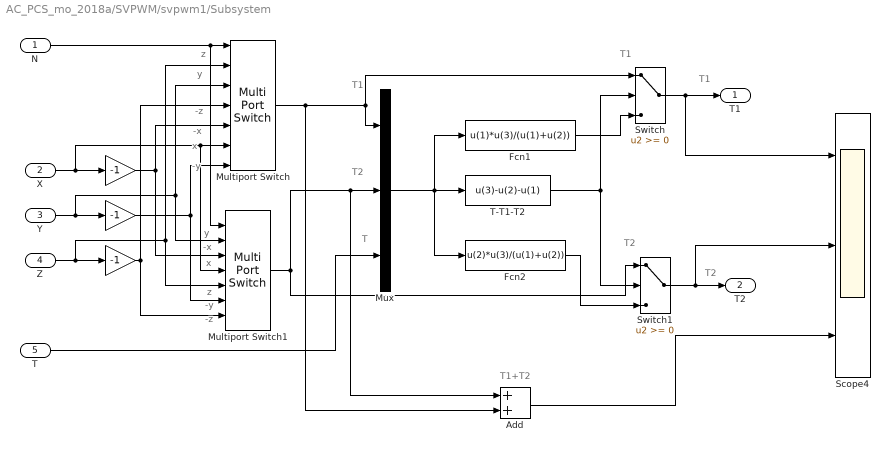
== system AC_PCS_mo_2018a/SVPWM/svpwm1/Subsystem ==
  note: T1
  note: T2
  note: T1+T2
  note: z
  note: y
  note: -z
  note: -x
  note: x
  note: -y
  note: y
  note: -x
  note: x
  note: z
  note: -y
  note: -z
  note: T1
  note: T2
  note: T
  note: T1
  note: T2
  N : Inport
  X : Inport  Port=2
  Y : Inport  Port=3
  Z : Inport  Port=4
  T : Inport  Port=5
  " " : Gain  Gain=-1
  "  " : Gain  Gain=-1
  "    " : Gain  Gain=-1
  Add : Sum
  Fcn1 : Fcn  Expr=u(1)*u(3)/(u(1)+u(2))
  Fcn2 : Fcn  Expr=u(2)*u(3)/(u(1)+u(2))
  Multiport Switch : MultiPortSwitch  Inputs=6  DiagnosticForDefault=None
  Multiport Switch1 : MultiPortSwitch  Inputs=6  DiagnosticForDefault=None
  Mux : Mux  Inputs=3
  Scope4 : Scope  NumInputPorts=3
  Switch : Switch
  Switch1 : Switch
  T-T1-T2 : Fcn  Expr=u(3)-u(2)-u(1)
  T1 : Outport
  T2 : Outport  Port=2
  wires:
  N/1 -> Multiport Switch1/1, Multiport Switch/1
  X/1 -> Multiport Switch1/4, Multiport Switch/6, " "/1
  Y/1 -> Multiport Switch1/2, Multiport Switch/3, "  "/1
  Z/1 -> Multiport Switch1/5, Multiport Switch/2, "    "/1
  "    "/1 -> Multiport Switch1/7, Multiport Switch/4
  "  "/1 -> Multiport Switch/7, Multiport Switch1/6
  " "/1 -> Multiport Switch/5, Multiport Switch1/3
  Multiport Switch/1 -> Mux/1, Switch/1, Add/2
  Multiport Switch1/1 -> Mux/2, Add/1, Switch1/1
  T/1 -> Mux/3
  Mux/1 -> T-T1-T2/1, Fcn1/1, Fcn2/1
  T-T1-T2/1 -> Switch/2, Switch1/2
  Fcn1/1 -> Switch/3
  Fcn2/1 -> Switch1/3
  Switch/1 -> T1/1, Scope4/1
  Switch1/1 -> T2/1, Scope4/2
  Add/1 -> Scope4/3

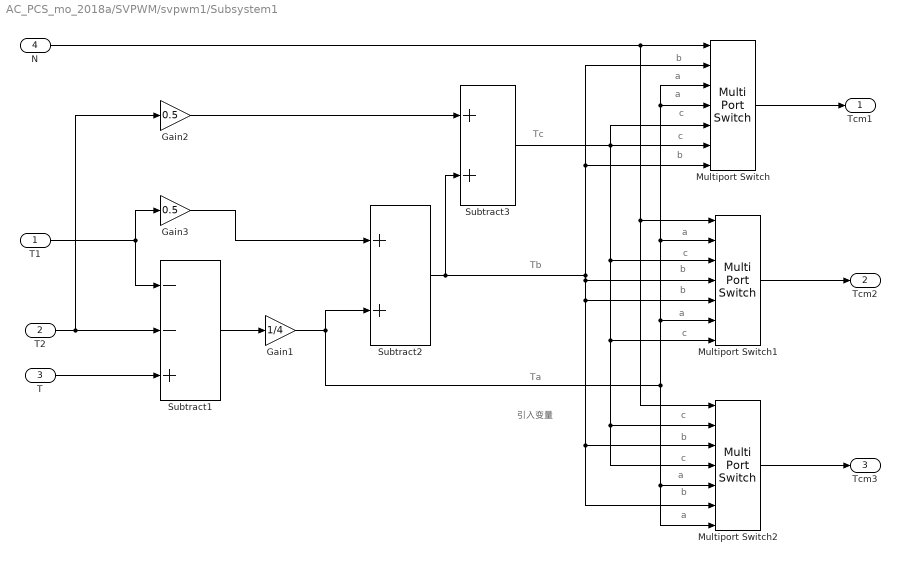
== system AC_PCS_mo_2018a/SVPWM/svpwm1/Subsystem1 ==
  note: 引入变量
  note: Ta
  note: Tb
  note: Tc
  note: b
  note: a
  note: a
  note: c
  note: c
  note: b
  note: a
  note: c
  note: b
  note: b
  note: a
  note: c
  note: c
  note: b
  note: c
  note: a
  note: b
  note: a
  T1 : Inport
  T2 : Inport  Port=2
  T : Inport  Port=3
  N : Inport  Port=4
  Gain1 : Gain  Gain=1/4
  Gain2 : Gain  Gain=0.5
  Gain3 : Gain  Gain=0.5
  Multiport Switch : MultiPortSwitch  Inputs=6  DiagnosticForDefault=None
  Multiport Switch1 : MultiPortSwitch  Inputs=6  DiagnosticForDefault=None
  Multiport Switch2 : MultiPortSwitch  Inputs=6  DiagnosticForDefault=None
  Subtract1 : Sum  Inputs=--+
  Subtract2 : Sum
  Subtract3 : Sum
  Tcm1 : Outport
  Tcm2 : Outport  Port=2
  Tcm3 : Outport  Port=3
  wires:
  T2/1 -> Gain2/1, Subtract1/2
  T/1 -> Subtract1/3
  T1/1 -> Gain3/1, Subtract1/1
  Gain3/1 -> Subtract2/1
  Subtract1/1 -> Gain1/1
  Gain1/1 -> Subtract2/2, Multiport Switch/3, Multiport Switch/4, Multiport Switch1/2, Multiport Switch1/6, Multiport Switch2/5, Multiport Switch2/7
  Subtract2/1 -> Subtract3/2, Multiport Switch/2, Multiport Switch/7, Multiport Switch1/4, Multiport Switch1/5, Multiport Switch2/3, Multiport Switch2/6
  Gain2/1 -> Subtract3/1
  N/1 -> Multiport Switch/1, Multiport Switch2/1, Multiport Switch1/1
  Multiport Switch/1 -> Tcm1/1
  Multiport Switch1/1 -> Tcm2/1
  Multiport Switch2/1 -> Tcm3/1
  Subtract3/1 -> Multiport Switch/5, Multiport Switch/6, Multiport Switch1/3, Multiport Switch1/7, Multiport Switch2/2, Multiport Switch2/4

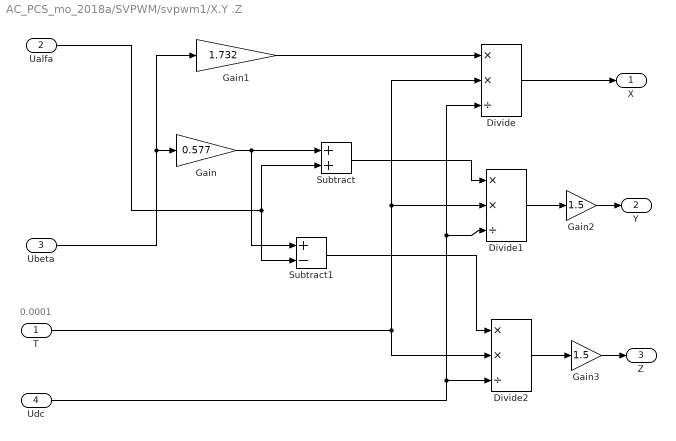
== system AC_PCS_mo_2018a/SVPWM/svpwm1/X.Y .Z ==
  note: 0.0001
  T : Inport
  Ualfa : Inport  Port=2
  Ubeta : Inport  Port=3
  Udc : Inport  Port=4
  Divide : Product  Inputs=**/
  Divide1 : Product  Inputs=**/
  Divide2 : Product  Inputs=**/
  Gain : Gain  Gain=0.577
  Gain1 : Gain  Gain=1.732
  Gain2 : Gain  Gain=1.5
  Gain3 : Gain  Gain=1.5
  Subtract : Sum
  Subtract1 : Sum  Inputs=+-
  X : Outport
  Y : Outport  Port=2
  Z : Outport  Port=3
  wires:
  Gain/1 -> Subtract/1, Subtract1/1
  Gain1/1 -> Divide/1
  T/1 -> Divide1/2, Divide/2, Divide2/2
  Udc/1 -> Divide2/3, Divide1/3, Divide/3
  Ualfa/1 -> Subtract1/2, Subtract/2
  Subtract/1 -> Divide1/1
  Subtract1/1 -> Divide2/1
  Divide/1 -> X/1
  Divide1/1 -> Gain2/1
  Divide2/1 -> Gain3/1
  Gain2/1 -> Y/1
  Gain3/1 -> Z/1
  Ubeta/1 -> Gain1/1, Gain/1

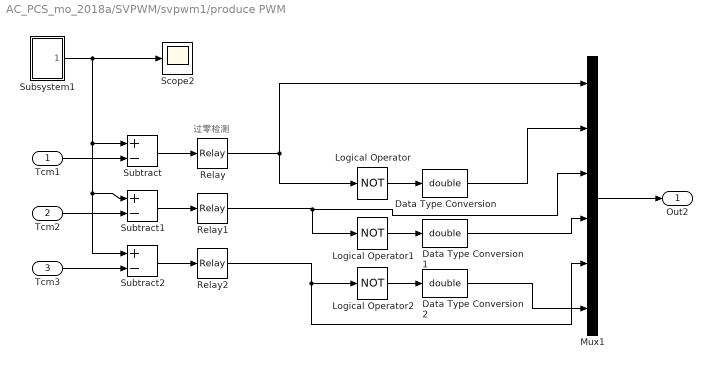
== system AC_PCS_mo_2018a/SVPWM/svpwm1/produce PWM ==
  note: 过零检测
  Tcm1 : Inport
  Tcm2 : Inport  Port=2
  Tcm3 : Inport  Port=3
  Data Type Conversion : DataTypeConversion  OutDataTypeStr=double
  Data Type Conversion1 : DataTypeConversion  OutDataTypeStr=double
  Data Type Conversion2 : DataTypeConversion  OutDataTypeStr=double
  Logical Operator : Logic  Operator=NOT  AllPortsSameDT=off
  Logical Operator1 : Logic  Operator=NOT  AllPortsSameDT=off
  Logical Operator2 : Logic  Operator=NOT  AllPortsSameDT=off
  Mux1 : Mux  Inputs=6
  Relay : Relay
  Relay1 : Relay
  Relay2 : Relay
  Scope2 : Scope
  Subsystem1 : Subsystem  AncestorBlock=Mylibrary/Subsystem2/produce PWM/Subsystem1
  Subtract : Sum  Inputs=+-
  Subtract1 : Sum  Inputs=+-
  Subtract2 : Sum  Inputs=+-
  Out2 : Outport
  wires:
  Subtract/1 -> Relay/1
  Subtract1/1 -> Relay1/1
  Subtract2/1 -> Relay2/1
  Subsystem1/1(Out1) -> Subtract/1, Subtract2/1, Subtract1/1, Scope2/1
  Tcm1/1 -> Subtract/2
  Tcm2/1 -> Subtract1/2
  Tcm3/1 -> Subtract2/2
  Logical Operator1/1 -> Data Type Conversion1/1
  Logical Operator2/1 -> Data Type Conversion2/1
  Logical Operator/1 -> Data Type Conversion/1
  Relay/1 -> Logical Operator/1, Mux1/1
  Relay1/1 -> Mux1/3, Logical Operator1/1
  Relay2/1 -> Mux1/5, Logical Operator2/1
  Mux1/1 -> Out2/1
  Data Type Conversion/1 -> Mux1/2
  Data Type Conversion1/1 -> Mux1/4
  Data Type Conversion2/1 -> Mux1/6

== system AC_PCS_mo_2018a/SVPWM/svpwm1/produce PWM/Subsystem1 ==
  note: 三角波最大值T/2
  Constant : Constant
  Integrator : Integrator
  Pulse Generator : DiscretePulseGenerator  PulseType=Time based  Amplitude=2  Period=0.0001  PulseWidth=50
  Scope : Scope  NumInputPorts=2
  Scope2 : Scope
  Sum : Sum  Inputs=|+-
  Out1 : Outport
  wires:
  Integrator/1 -> Scope/2, Out1/1
  Sum/1 -> Scope/1, Integrator/1
  Constant/1 -> Sum/2
  Pulse Generator/1 -> Scope2/1, Sum/1
